simulink model "Generic_sedan"  (R2023b)
settings: Solver=VariableStepAuto  StartTime=0.0  StopTime=26  FixedStep=0.001  MaxStep=0.01  RelTol=1e-4
InitFcn:
  | A = readmatrix(['data' filesep 'A.dat']);
  | B = readmatrix(['data' filesep 'B.dat']);
  | C = readmatrix(['data' filesep 'C.dat']);
  | D = readmatrix(['data' filesep 'D.dat']);
  | 
  | Z0 = readmatrix(['data' filesep 'Z0.dat']);
  | m = readmatrix(['data' filesep 'mass.dat']);
  | IG = readmatrix(['data' filesep 'IG.dat']);
  | 
  | z = readmatrix(['data' filesep 'z.dat']);
  | l = readmatrix(['data' filesep 'l.dat']);
  | fbf = readmatrix(['data' filesep 'brake.dat']);
libraries: simulink x10, matrix_library x2, slpidlib x1
(part 1 of 2)
settings Model: Creator=minaker  LastModifiedBy=minaker
settings SimscapeCC: EditingMode=Restricted

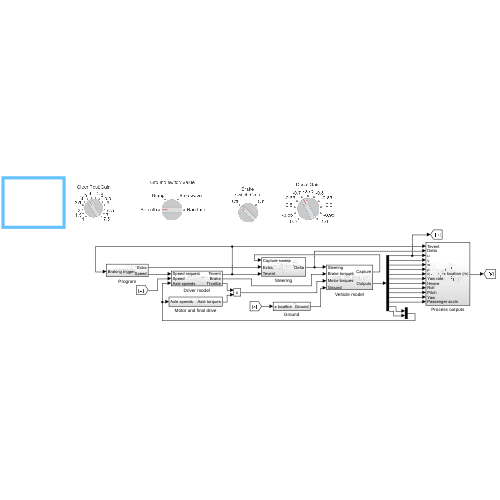
[thumbnail: Simulink's stored preview of the top-level diagram]
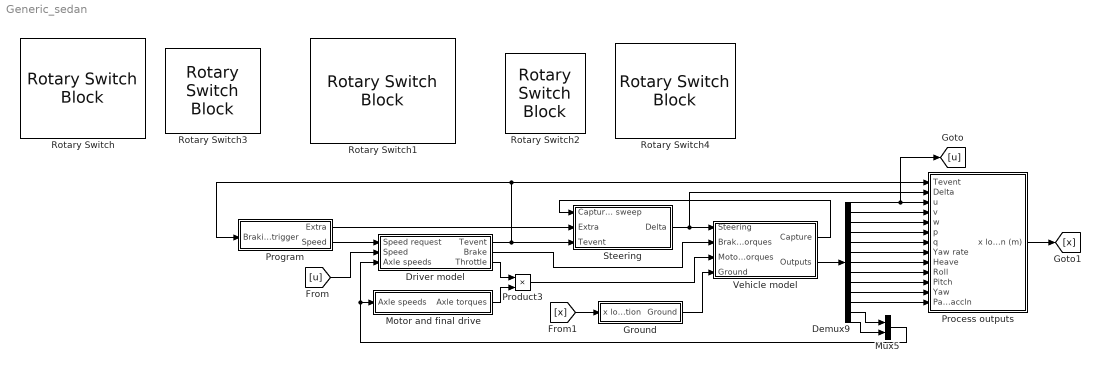
== system Generic_sedan ==
  Demux9 : Demux  Outputs=13
  Driver model : Subsystem
  Ground : Subsystem
  Motor and final drive : Subsystem
  Mux5 : Mux  Inputs=2
  Process outputs : Subsystem
  Product3 : Product
  Program : Subsystem
  Rotary Switch{,1..4} (5 alike) : RotarySwitchBlock
  Steering : Subsystem
  Vehicle model : Subsystem
  wires:
  Product3/1 -> Vehicle model/3(Motor torques)
  Vehicle model/2(Outputs) -> Demux9/1
  Demux9/12 -> Mux5/1
  Demux9/13 -> Mux5/2
  Motor and final drive/1(Axle torques) -> Product3/2
  Demux9/2 -> Process outputs/4(v)
  Demux9/1 -> [u], Process outputs/3(u)
  Demux9/10 -> Process outputs/12(Yaw)
  Driver model/2(Brake) -> Vehicle model/2(Brake torques)
  Driver model/3(Throttle) -> Product3/1
  Demux9/6 -> Process outputs/8(Yaw rate)
  Demux9/8 -> Process outputs/10(Roll)
  Demux9/9 -> Process outputs/11(Pitch)
  Demux9/7 -> Process outputs/9(Heave)
  Demux9/11 -> Process outputs/13(Passenger accln)
  Steering/1(Delta) -> Process outputs/2(Delta), Vehicle model/1(Steering)
  Vehicle model/1(Capture) -> Steering/1(Capture sweep)
  Demux9/3 -> Process outputs/5(w)
  Demux9/4 -> Process outputs/6(p)
  Demux9/5 -> Process outputs/7(q)
  [u] -> Driver model/2(Speed)
  Process outputs/1(x location (m)) -> [x]
  Driver model/1(Tevent) -> Program/1(Braking trigger), Process outputs/1(Tevent), Steering/3(Tevent)
  Mux5/1 -> Driver model/3(Axle speeds), Motor and final drive/1(Axle speeds)
  Program/1(Extra) -> Steering/2(Extra)
  Program/2(Speed) -> Driver model/1(Speed request)
  [x] -> Ground/1(x location)
  Ground/1(Ground) -> Vehicle model/4(Ground)

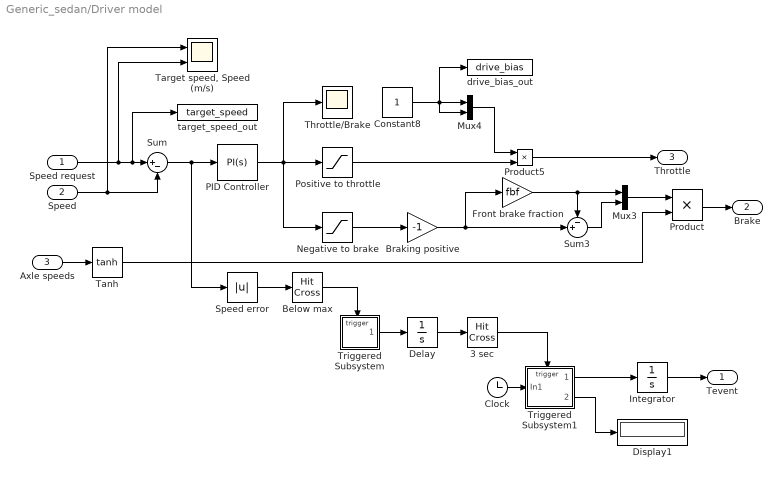
== system Generic_sedan/Driver model ==
  Speed request : Inport
  Speed : Inport  Port=2
  Axle speeds : Inport  Port=3
  3 sec : HitCross  HitCrossingOffset=3  HitCrossingDirection=rising
  Below max : HitCross  HitCrossingOffset=0.1  HitCrossingDirection=falling
  Braking positive : Gain  Gain=-1
  Clock : Clock
  Constant8 : Constant
  Delay : Integrator
  Display1 : Display
  Front brake fraction : Gain  Gain=fbf
  Integrator : Integrator
  Mux3 : Mux  Inputs=2
  Mux4 : Mux  Inputs=2
  Negative to brake : Saturate  UpperLimit=0  LowerLimit=-Inf
  PID Controller : slpidlib/PID Controller  Controller=PI  Form=Parallel  TimeDomain=Continuous-time  UseExternalTs=off  SampleTime=-1  IntegratorMethod=Forward Euler  FilterMethod=Forward Euler  ControllerParametersSource=internal  P=0.75  I=0.0075  UseKiTs=off  D=0.2  N=100  UseFilter=on  TunerSelectOption=Transfer Function Based (PID Tuner App)  InitialConditionSource=internal  InitialConditionForIntegrator=0  InitialConditionForFilter=0  DifferentiatorICPrevScaledInput=0  ExternalReset=none  TrackingMode=off  Kt=1  LimitOutput=on  SatLimitsSource=internal  UpperSaturationLimit=1  LowerSaturationLimit=-1  LinearizeAsGain=on  AntiWindupMode=clamping  Kb=1  LimitIntegrator=off  UpperIntegratorSaturationLimit=inf  LowerIntegratorSaturationLimit=-inf  POutMin=[]  POutMax=[]  IOutMin=[]  IOutMax=[]  DOutMin=[]  DOutMax=[]  NOutMin=[]  NOutMax=[]  SumOutMin=[]  SumOutMax=[]  SaturationOutMin=[]  SaturationOutMax=[]  PParamMin=[]  PParamMax=[]  IParamMin=[]  IParamMax=[]  DParamMin=[]  DParamMax=[]  NParamMin=[]  NParamMax=[]  KbParamMin=[]  KbParamMax=[]  KtParamMin=[]  KtParamMax=[]  KbOutMin=[]  KbOutMax=[]  KtOutMin=[]  KtOutMax=[]  IntegratorOutMin=[]  IntegratorOutMax=[]  FilterOutMin=[]  FilterOutMax=[]  SumI1OutMin=[]  SumI1OutMax=[]  SumI2OutMin=[]  SumI2OutMax=[]  SumI3OutMin=[]  SumI3OutMax=[]  SumI4OutMin=[]  SumI4OutMax=[]  SumDOutMin=[]  SumDOutMax=[]  DifferentiatorOutMin=[]  DifferentiatorOutMax=[]  FilterDiffOutCoefMin=[]  FilterDiffOutCoefMax=[]  ReciprocalOutMin=[]  ReciprocalOutMax=[]  SumDenOutMin=[]  SumDenOutMax=[]  SumNumOutMin=[]  SumNumOutMax=[]  DivideOutMin=[]  DivideOutMax=[]  UdiffTsProdOutMin=[]  UdiffTsProdOutMax=[]  NTsProdOutMin=[]  NTsProdOutMax=[]  UintegralTsProdOutMin=[]  UintegralTsProdOutMax=[]  UngainTsProdOutMin=[]  UngainTsProdOutMax=[]  ClampingZeroOutDataTypeStr=Inherit: Inherit via back propagation  ClampingZeroOutMin=[]  ClampingZeroOutMax=[]  FilterDenConstantOutDataTypeStr=Inherit: Inherit via back propagation  FilterDenConstantOutMin=[]  FilterDenConstantOutMax=[]  PCopyOutDataTypeStr=Inherit: Inherit via back propagation  PCopyOutMin=[]  PCopyOutMax=[]  NCopyOutDataTypeStr=Inherit: Inherit via back propagation  NCopyOutMin=[]  NCopyOutMax=[]  IntegratorContinuousStateAttributes=''  IntegratorStateMustResolveToSignalObject=off  IntegratorRTWStateStorageClass=Auto  FilterContinuousStateAttributes=''  FilterStateMustResolveToSignalObject=off  FilterRTWStateStorageClass=Auto  ParallelPVariant=InternalParameters  IdealPVariant=Disabled  IVariant=InternalParameters  DVariant=Disabled  IntegratorVariant=Continuous  SatVariant=Enabled  AWVariant=ContClampingParallel  PCopyVariant=Disabled  TRVariant=Disabled  FdbkBlocksVariant=Forward  IdealPFdbkVariant=Disabled  SatFdbkVariant=Disabled  DerivativeFilterVariant=Disabled  NVariant=Disabled  NCopyVariant=Disabled_SignalSpec  FilterICVariant=Disabled  IntegratorICVariant=InternalICs  ExternalResetVariant=Disabled  TRSumVariant=Passthrough  SumFdbkVariant=Disabled  SumVariant=Sum_PI  TsampFilterVariant=InternalTs  TsampNgainVariant=Passthrough  TsampIntegralVariant=Disabled_SignalSpec  ExternalSaturationOutDataTypeStr=Inherit: Same as second input
  Positive to throttle : Saturate  UpperLimit=Inf  LowerLimit=0
  Product : Product
  Product5 : Product
  Speed error : Abs  SaturateOnIntegerOverflow=off
  Sum : Sum  Inputs=|+-
  Sum3 : Sum  Inputs=-+|
  Tanh : Trigonometry  Operator=tanh
  "Target speed, Speed (m/s)" : Scope  NumInputPorts=2
  Throttle/Brake : Scope
  Triggered Subsystem : Subsystem  TreatAsAtomicUnit=on
  Triggered Subsystem1 : Subsystem  TreatAsAtomicUnit=on
  drive_bias_out : ToWorkspace  VariableName=drive_bias  SaveFormat=Timeseries  SampleTime=-1
      settings: Decimation=3
  target_speed_out : ToWorkspace  VariableName=target_speed  SaveFormat=Timeseries  SampleTime=-1
      settings: Decimation=3
  Tevent : Outport
  Brake : Outport  Port=2
  Throttle : Outport  Port=3
  wires:
  Product5/1 -> Throttle/1
  Speed/1 -> "Target speed, Speed (m/s)"/1, Sum/2
  Mux4/1 -> Product5/1
  Positive to throttle/1 -> Product5/2
  Constant8/1 -> drive_bias_out/1, Mux4/1, Mux4/2
  PID Controller/1 -> Throttle/Brake/1, Negative to brake/1, Positive to throttle/1
  Braking positive/1 -> Front brake fraction/1, Sum3/2
  Speed request/1 -> target_speed_out/1, Sum/1, "Target speed, Speed (m/s)"/2
  Sum3/1 -> Mux3/2
  Front brake fraction/1 -> Mux3/1, Sum3/1
  Negative to brake/1 -> Braking positive/1
  Mux3/1 -> Product/1
  Sum/1 -> Speed error/1, PID Controller/1
  Speed error/1 -> Below max/1
  Triggered Subsystem/1(Out1) -> Delay/1
  Below max/1 -> Triggered Subsystem/Trigger
  3 sec/1 -> Triggered Subsystem1/Trigger
  Delay/1 -> 3 sec/1
  Triggered Subsystem1/1(Out1) -> Integrator/1
  Triggered Subsystem1/2(Start time) -> Display1/1
  Clock/1 -> Triggered Subsystem1/1(In1)
  Integrator/1 -> Tevent/1
  Tanh/1 -> Product/2
  Axle speeds/1 -> Tanh/1
  Product/1 -> Brake/1

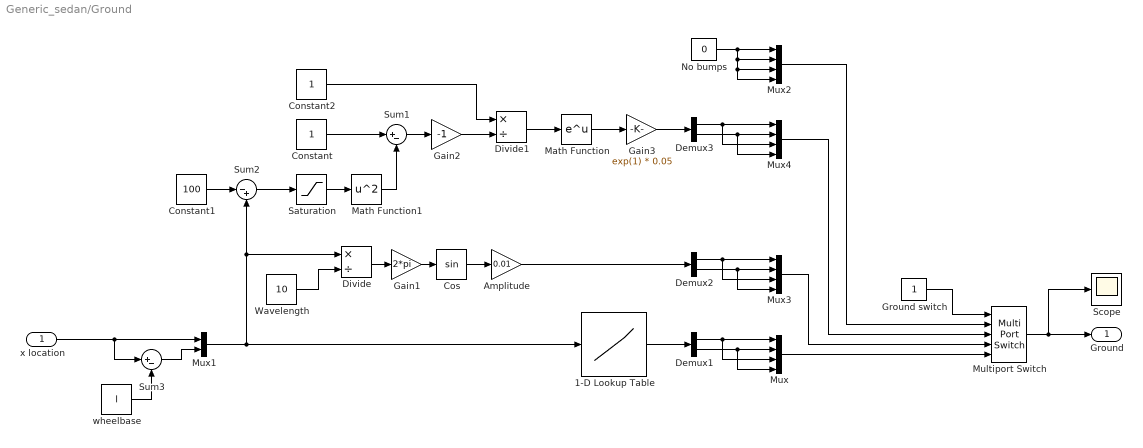
== system Generic_sedan/Ground ==
  x location : Inport
  1-D Lookup Table : Lookup_n-D  NumberOfTableDimensions=1  BreakpointsForDimension1=z(:,1)  Table=z(:,2)  ExtrapMethod=Clip  InternalRulePriority=Speed  RndMeth=Simplest
  Amplitude : Gain  Gain=0.01
  Constant : Constant
  Constant1 : Constant  Value=100
  Constant2 : Constant
  Cos : Trigonometry
  Demux1 : Demux  Outputs=2
  Demux2 : Demux  Outputs=2
  Demux3 : Demux  Outputs=2
  Divide : Product  Inputs=*/
  Divide1 : Product  Inputs=*/
  Gain1 : Gain  Gain=2*pi
  Gain2 : Gain  Gain=-1
  Gain3 : Gain  Gain=exp(1) * 0.05
  Ground switch : Constant
  Math Function : Math
  Math Function1 : Math  Operator=square
  Multiport Switch : MultiPortSwitch  Inputs=4  SaturateOnIntegerOverflow=off  InputSameDT=off
  Mux{,2..4} (4 alike) : Mux
  Mux1 : Mux  Inputs=2
  No bumps : Constant  Value=0
  Saturation : Saturate  UpperLimit=1  LowerLimit=-1
  Scope : Scope
  Sum1 : Sum  Inputs=|+-
  Sum2 : Sum  Inputs=|-+
  Sum3 : Sum  Inputs=|+-
  Wavelength : Constant  Value=10
  wheelbase : Constant  Value=l
  Ground : Outport
  wires:
  Mux2/1 -> Multiport Switch/2
  Multiport Switch/1 -> Scope/1, Ground/1
  Demux1/2 -> Mux/4, Mux/2
  Demux1/1 -> Mux/3, Mux/1
  wheelbase/1 -> Sum3/2
  Sum3/1 -> Mux1/2
  1-D Lookup Table/1 -> Demux1/1
  Ground switch/1 -> Multiport Switch/1
  Mux/1 -> Multiport Switch/5
  x location/1 -> Sum3/1, Mux1/1
  No bumps/1 -> Mux2/3, Mux2/4, Mux2/2, Mux2/1
  Amplitude/1 -> Demux2/1
  Mux1/1 -> Divide/1, Sum2/2, 1-D Lookup Table/1
  Demux2/2 -> Mux3/4, Mux3/2
  Demux2/1 -> Mux3/3, Mux3/1
  Mux3/1 -> Multiport Switch/4
  Divide/1 -> Gain1/1
  Gain1/1 -> Cos/1
  Wavelength/1 -> Divide/2
  Cos/1 -> Amplitude/1
  Gain2/1 -> Divide1/2
  Divide1/1 -> Math Function/1
  Constant/1 -> Sum1/1
  Math Function1/1 -> Sum1/2
  Sum1/1 -> Gain2/1
  Saturation/1 -> Math Function1/1
  Constant1/1 -> Sum2/1
  Sum2/1 -> Saturation/1
  Math Function/1 -> Gain3/1
  Constant2/1 -> Divide1/1
  Gain3/1 -> Demux3/1
  Demux3/1 -> Mux4/3, Mux4/1
  Demux3/2 -> Mux4/4, Mux4/2
  Mux4/1 -> Multiport Switch/3

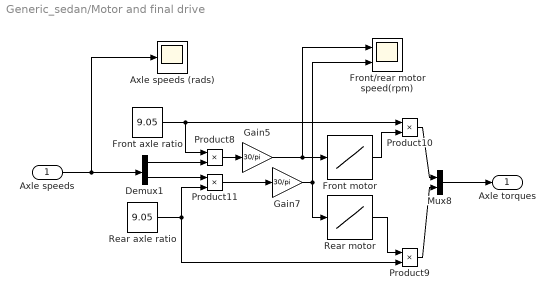
== system Generic_sedan/Motor and final drive ==
  Axle speeds : Inport
  Axle speeds (rads) : Scope
  Demux1 : Demux  Outputs=2
  Front axle ratio : Constant  Value=9.05
  Front motor : Lookup_n-D  NumberOfTableDimensions=1  BreakpointsForDimension1=[0;50;100;150;200;250;300;350;400;450;500;550;600;650;700;750;800;850;900;950;1000;1050;1100;1150;1200;1250;1300;1350;1400;1450;1500;1550;1600;1650;1700;1750;1800;1850;1900;1950;2000;2050;2100;2150;2200;2250;2300;2350;2400;2450;2500;2550;2600;2650;2700;2750;2800;2850;2900;2950;3000;3050;3100;3150;3200;3250;3300;3350;3400;3450;3500;3550;3600;3650;3700;3750;3800;3850;3900;3950;4000;4050;4100;4150;4200;4250;4300;4350;4400;4450;4500;4550;4600;4650;4700;4750;4800;4850;4900;4950;5000;5050;5100;5150;5200;5250;5300;5350;5400;5450;5500;5550;5600;5650;5700;5750;5800;5850;5900;5950;6000;6050;6100;6150;6200;6250;6300;6350;6400;6450;6500;6550;6600;6650;6700;6750;6800;6850;6900;6950;7000;7050;7100;7150;7200;7250;7300;7350;7400;7450;7500;7550;7600;7650;7700;7750;7800;7850;7900;7950;8000;8050;8100;8150;8200;8250;8300;8350;8400;8450;8500;8550;8600;8650;8700;8750;8800;8850;8900;8950;9000;9050;9100;9150;9200;9250;9300;9350;9400;9450;9500;9550;9600;9650;9700;9750;9800;9850;9900;9950;10000;10050;10100;10150;10200;10250;10300;10350;10400;10450;10500;10550;10600;10650;10700;10750;10800;10850;10900;10950;11000;11050;11100;11150;11200;11250;11300;11350;11400;11450;11500;11550;11600;11650;11700;11750;11800;11850;11900;11950;12000;12050;12100;12150;12200;12250;12300;12350;12400;12450;12500;12550;12600;12650;12700;12750;12800;12850;12900;12950;13000;13050;13100;13150;13200;13250;13300;13350;13400;13450;13500;13550;13600;13650;13700;13750;13800]  Table=[151.278471649211;150.863507782483;150.857645204683;150.851798439641;150.845961214183;150.840130739586;150.834305445898;150.828484331262;150.822666703624;150.816852057881;150.811040010119;150.805230259282;150.799422563368;150.793616723888;150.787812575288;150.782009977530;150.776208810713;150.770408971108;150.764610368151;150.758812922132;150.753016562399;150.747221225919;150.741426856141;150.735633402060;150.729840817460;150.724049060281;150.718258092094;150.712467877664;150.706678384571;150.700889582896;150.695101444949;150.689313945031;150.683527059236;150.677740765271;150.671955042299;150.666169870810;150.660385232498;150.654601110154;150.648817487573;150.643034349475;150.637251681422;150.631469469760;150.625687701550;150.619906364522;150.614125447022;150.608344937967;150.602564826808;150.596785103490;150.591005758422;150.585226782442;150.579448166795;150.573669903103;150.567891983343;150.562114399825;150.556337145175;150.550560212312;150.544783594433;150.539007284998;150.533231277717;150.527455566531;150.521680145605;150.515905009314;150.510130152233;150.504355569124;150.498581254931;148.374181079972;146.125974258770;143.945037424496;141.828191440898;139.772684341068;137.775894243506;135.835157562690;133.948829662349;132.113904887137;130.328575497099;128.590978243296;126.898873510717;125.250831781071;123.645086677358;122.079845291043;120.553855681789;119.065531893495;117.613516943143;116.196631674882;114.813197353996;113.462607953756;112.143116898742;110.854289029982;109.594402325692;108.362997543078;107.158884499023;105.981325021586;104.829358289475;103.702163956374;102.598944505611;101.518963997732;100.461458577429;99.4257696628103;98.4112032057036;97.4169803632393;96.4428468494649;95.4879934255911;94.5519655023934;93.6336039738249;92.7339362228427;91.8503667621564;90.9842571556953;90.1335231457530;89.2993699380107;88.4796659256438;87.6757465870287;86.8854186202727;86.1095497053428;85.3480053387293;84.5988715272067;83.8638251758735;83.1403184969489;82.4296640384837;81.7310399176694;81.0447873302831;80.3688805105759;79.7051959749083;79.0517449603443;78.4086231766840;77.7762824954103;77.1545523243600;76.5415929088006;75.9390023745799;75.3457153739749;74.7616213898289;74.1870080607537;73.6201508895266;73.0629516796206;72.5131001669698;71.9719338669643;71.4393535756975;70.9134865309499;70.3963184515362;69.8864581840491;69.3829019088306;68.8873785972233;68.3994010157060;67.9178864974784;67.4421538676144;66.9737815819947;66.5124360742594;66.0562807895463;65.6074841358173;65.1635947359257;64.7268069675545;64.2947231500399;63.8694815701027;63.4487227952091;63.0345689138391;62.6255122413869;62.2206415044942;61.8223298316254;61.4279939494809;61.0397435640339;60.6561280103982;60.2761819776827;59.9023223995399;59.5328468246745;59.1667632052020;58.8065098220250;58.4504077906492;58.0974490866022;57.7500709024121;57.4066274669585;57.0660939915105;56.7309147606174;56.3994683410035;56.0707202646022;55.7471069493456;55.4262052260204;55.1099727704398;54.7971666570846;54.4867411788298;54.1811164617496;53.8787500903933;53.5795924172299;53.2825709746378;52.9902784666275;52.7010368836716;52.4137990680552;52.1309413888743;51.8509908230479;51.5739038180854;51.2985649381260;51.0275936092540;50.7593508293397;50.4927991289585;50.2302556320192;49.9703169896832;49.7119478679885;49.4574468745715;49.2054333900219;48.9558725933389;48.7076241958030;48.4632837399324;48.2212850899552;47.9815973534268;47.7430784882541;47.5082121649214;47.2756519874389;47.0442958892288;46.8163352461487;46.5904893858102;46.3667271851825;46.1439110744480;45.9245721439951;45.7072299260645;45.4918575830820;45.2773233799879;45.0661281374574;44.8568211134734;44.6493778189262;44.4437738063396;44.2387987606263;44.0371626899314;43.8372897474568;43.6391585877190;43.4416546749887;43.2472080094171;43.0544327298518;42.8633080852959;42.6738128625357;42.4847391415345;42.2987511504260;42.1143278668312;41.9314509531562;41.7501004959835;41.5690724994407;41.3910035521333;41.2144025457871 ...(+714 chars)]  InternalRulePriority=Speed  RndMeth=Simplest
  Front/rear motor speed(rpm) : Scope  NumInputPorts=2
  Gain5 : Gain  Gain=30/pi
  Gain7 : Gain  Gain=30/pi
  Mux8 : Mux  Inputs=2
  Product{8..11} (4 alike) : Product
  Rear axle ratio : Constant  Value=9.05
  Rear motor : Lookup_n-D  NumberOfTableDimensions=1  BreakpointsForDimension1=[0;50;100;150;200;250;300;350;400;450;500;550;600;650;700;750;800;850;900;950;1000;1050;1100;1150;1200;1250;1300;1350;1400;1450;1500;1550;1600;1650;1700;1750;1800;1850;1900;1950;2000;2050;2100;2150;2200;2250;2300;2350;2400;2450;2500;2550;2600;2650;2700;2750;2800;2850;2900;2950;3000;3050;3100;3150;3200;3250;3300;3350;3400;3450;3500;3550;3600;3650;3700;3750;3800;3850;3900;3950;4000;4050;4100;4150;4200;4250;4300;4350;4400;4450;4500;4550;4600;4650;4700;4750;4800;4850;4900;4950;5000;5050;5100;5150;5200;5250;5300;5350;5400;5450;5500;5550;5600;5650;5700;5750;5800;5850;5900;5950;6000;6050;6100;6150;6200;6250;6300;6350;6400;6450;6500;6550;6600;6650;6700;6750;6800;6850;6900;6950;7000;7050;7100;7150;7200;7250;7300;7350;7400;7450;7500;7550;7600;7650;7700;7750;7800;7850;7900;7950;8000;8050;8100;8150;8200;8250;8300;8350;8400;8450;8500;8550;8600;8650;8700;8750;8800;8850;8900;8950;9000;9050;9100;9150;9200;9250;9300;9350;9400;9450;9500;9550;9600;9650;9700;9750;9800;9850;9900;9950;10000;10050;10100;10150;10200;10250;10300;10350;10400;10450;10500;10550;10600;10650;10700;10750;10800;10850;10900;10950;11000;11050;11100;11150;11200;11250;11300;11350;11400;11450;11500;11550;11600;11650;11700;11750;11800;11850;11900;11950;12000;12050;12100;12150;12200;12250;12300;12350;12400;12450;12500;12550;12600;12650;12700;12750;12800;12850;12900;12950;13000;13050;13100;13150;13200;13250;13300;13350;13400;13450;13500;13550;13600;13650;13700;13750;13800]  Table=[432.243928408188;430.974439582432;430.956179022406;430.937971427874;430.919796209269;430.901644104877;430.883509858563;430.865390095315;430.847282471915;430.829185270798;430.811097181604;430.793017173390;430.774944414988;430.756878222831;430.738818025389;430.720763338111;430.702713745266;430.684668886477;430.666628446533;430.648592147528;430.630559742721;430.612531011656;430.594505756247;430.576483797589;430.558464973357;430.540449135636;430.522436149121;430.504425889595;430.486418242650;430.468413102584;430.450410371463;430.432409958315;430.414411778418;430.396415752698;430.378421807187;430.360429872554;430.342439883693;430.324451779352;430.306465501809;430.288480996581;430.270498212163;430.252517099794;430.234537613252;430.216559708658;430.198583344313;430.180608480534;430.162635079523;430.144663105232;430.126692523248;430.108723300689;430.090755406101;430.072788809376;430.054823481660;430.036859395286;430.018896523699;430.000934841393;429.982974323852;429.965014947491;429.947056689611;429.929099528346;429.911143442620;429.893188412107;429.875234417191;429.857281438932;429.839329459032;429.821378459799;427.981721433497;421.593724980700;415.393957153120;409.373720022615;403.525491314955;397.842014747280;392.316393278445;386.942169399268;381.713191334335;376.622937315821;371.667497699383;366.841160078948;362.137730929994;357.553828148806;353.084910683754;348.725261434143;344.472711529334;340.322323403211;336.270778863834;332.314595712636;328.450457205214;324.675146866800;320.985637221670;317.379016616004;313.852538681236;310.403848313197;307.030644702009;303.729239788566;300.498074173125;297.334940004498;294.237701043453;291.204256508991;288.232850000853;285.321365981808;282.468192927640;279.671478179448;276.929600964921;274.240964075862;271.604031735127;269.017326671512;266.479427359743;263.988965414691;261.544623132608;259.145131165270;256.789266322546;254.475849492834;252.203743675887;249.971852119045;247.779116552168;245.624515514459;243.507062767986;241.425805792333;239.379824355837;237.368229158974;235.390160545651;233.444787397876;231.531305336144;229.648936957453;227.796929383204;225.974553870265;224.181104888187;222.415899192137;220.678274919441;218.967590603395;217.283224394710;215.624573747959;213.991054310818;212.382098840968;210.797157691598;209.235697164105;207.697199156691;206.181161134820;204.687094611862;203.214525470400;201.762992987159;200.332049501511;198.921260102066;197.530202106113;196.158464161338;194.805646820932;193.471361175082;192.155229003378;190.856882259308;189.575962937981;188.312122535456;187.065021661250;185.834329552786;184.619725127149;183.420894478029;182.237532335583;181.069341668332;179.916031372645;178.777319974436;177.652931593355;176.542597603395;175.446056040499;174.363051394840;173.293334410585;172.236661892536;171.192796519340;170.161506663305;169.142566215623;168.135754417792;167.140855698028;166.157659512809;165.186077775014;164.225693601322;163.276412134865;162.338041949438;161.410395996382;160.493291527820;159.586549792313;158.689996323496;157.803460118424;156.926773874417;156.059775120300;155.202303824061;154.354203797618;153.515322248111;152.685509686281;151.864619837427;151.052509555544;150.249038739976;149.454070254761;148.667469850468;147.889106088577;147.118850267707;146.356576352747;145.602160905490;144.855483017336;144.116424244760;143.384868544377;142.660702212323;141.943813822632;141.234094168514;140.531436203406;139.835734983580;139.146887610424;138.464793172002;137.789352685506;137.120469035850;136.458046910424;135.801992734899;135.152214593453;134.508622146712;133.871126584102;133.239713675600;132.614175112303;131.994482703112;131.380554873391;130.772311558861;130.169674170608;129.572565560543;128.980909988777;128.394633087277;127.813661829509;127.237924489186;126.667350600028;126.101870893083;125.541417204238;124.985922291029;124.435319446649;123.889541580428;123.348555891353;122.812257815484;122.280602993833;121.753531285584;121.230982638504;120.712902960770 ...(+714 chars)]  InternalRulePriority=Speed  RndMeth=Simplest
  Axle torques : Outport
  wires:
  Front axle ratio/1 -> Product10/1, Product8/1
  Mux8/1 -> Axle torques/1
  Axle speeds/1 -> Demux1/1, Axle speeds (rads)/1
  Product8/1 -> Gain5/1
  Product10/1 -> Mux8/1
  Demux1/2 -> Product11/1
  Gain7/1 -> Rear motor/1, Front/rear motor speed(rpm)/2
  Rear axle ratio/1 -> Product9/2, Product11/2
  Demux1/1 -> Product8/2
  Rear motor/1 -> Product9/1
  Product11/1 -> Gain7/1
  Product9/1 -> Mux8/2
  Gain5/1 -> Front/rear motor speed(rpm)/1, Front motor/1
  Front motor/1 -> Product10/2

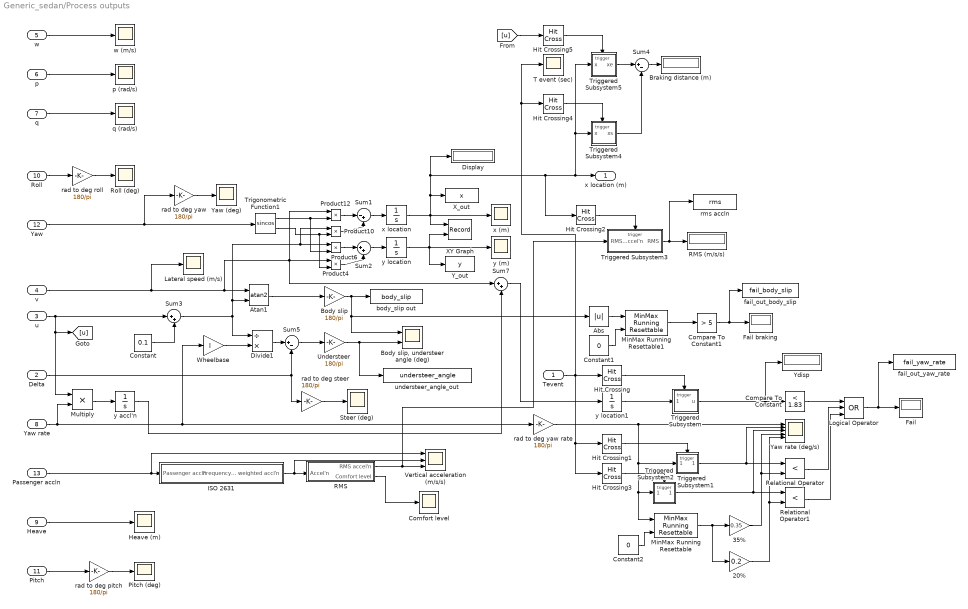
== system Generic_sedan/Process outputs ==
  Tevent : Inport
  Delta : Inport  Port=2
  u : Inport  Port=3
  v : Inport  Port=4
  w : Inport  Port=5
  p : Inport  Port=6
  q : Inport  Port=7
  Yaw rate : Inport  Port=8
  Heave : Inport  Port=9
  Roll : Inport  Port=10
  Pitch : Inport  Port=11
  Yaw : Inport  Port=12
  Passenger accln : Inport  Port=13
  20% : Gain  Gain=0.2
  35% : Gain  Gain=0.35
  Abs : Abs  SaturateOnIntegerOverflow=off
  Atan1 : Trigonometry  Operator=atan2
  Body slip : Gain  Gain=180/pi
  "Body slip, understeer angle (deg)" : Scope  NumInputPorts=2
  Braking distance (m) : Display
  Comfort level : Scope
  Compare To Constant : simulink/Logic and Bit Operations/Compare To Constant  relop=<  const=1.83  OutDataTypeStr=boolean
  Compare To Constant1 : simulink/Logic and Bit Operations/Compare To Constant  relop=>  const=5  OutDataTypeStr=boolean
  Constant : Constant  Value=0.1
  Constant1 : Constant  Value=0  OutDataTypeStr=boolean
  Constant2 : Constant  Value=0  OutDataTypeStr=boolean
  Display : Display
  Divide1 : Product  Inputs=/*
  Fail : Display
  Fail braking : Display
  Heave (m) : Scope
  Hit Crossing : HitCross  HitCrossingOffset=0.75/0.7  HitCrossingDirection=rising
  Hit Crossing1 : HitCross  HitCrossingOffset=1/0.7+0.5+1  HitCrossingDirection=rising
  Hit Crossing2 : HitCross  HitCrossingOffset=500  HitCrossingDirection=rising
  Hit Crossing3 : HitCross  HitCrossingOffset=1/0.7+0.5+1.75  HitCrossingDirection=rising
  Hit Crossing4 : HitCross  HitCrossingOffset=1e-6  HitCrossingDirection=rising
  Hit Crossing5 : HitCross  HitCrossingOffset=8/3.6  HitCrossingDirection=falling
  ISO 2631 : Subsystem
  Lateral speed (m/s) : Scope
  Logical Operator : Logic  Operator=OR  Inputs=3  AllPortsSameDT=off  OutDataTypeStr=boolean
  MinMax Running Resettable : simulink/Math Operations/MinMax Running Resettable  Function=min  vinit=0.0
  MinMax Running Resettable1 : simulink/Math Operations/MinMax Running Resettable  Function=max  vinit=0.0
  Multiply : Product  Inputs=**
  Pitch (deg) : Scope
  Product{4,6,10,12} (4 alike) : Product
  RMS : Subsystem
  RMS (m/s/s) : Display
  Relational Operator : RelationalOperator  Operator=<  OutDataTypeStr=boolean  RndMeth=Simplest  InputSameDT=off
  Relational Operator1 : RelationalOperator  Operator=<  OutDataTypeStr=boolean  RndMeth=Simplest  InputSameDT=off
  Roll (deg) : Scope
  Steer (deg) : Scope
  Sum1 : Sum  Inputs=|-+
  Sum2 : Sum  Inputs=|++
  Sum3 : Sum  Inputs=|++
  Sum4 : Sum  Inputs=|+-
  Sum5 : Sum  Inputs=|+-
  Sum7 : Sum  Inputs=|++
  T event (sec) : Scope
  Triggered Subsystem : Subsystem  TreatAsAtomicUnit=on
  Triggered Subsystem1 : Subsystem  TreatAsAtomicUnit=on
  Triggered Subsystem2 : Subsystem  TreatAsAtomicUnit=on
  Triggered Subsystem3 : Subsystem  TreatAsAtomicUnit=on
  Triggered Subsystem4 : Subsystem  TreatAsAtomicUnit=on
  Triggered Subsystem5 : Subsystem  TreatAsAtomicUnit=on
  Trigonometric Function1 : Trigonometry  Operator=sincos
  Understeer : Gain  Gain=180/pi
  Vertical acceleration (m/s/s) : Scope  NumInputPorts=3
  Wheelbase : Gain  Gain=l
  XY Graph : Record  FileSettingsInternal="{\"entries\":[{\"content\":{\"excelSettings\":{\"content\":{},\"type\":\"Streamout.ExcelSettings\"}},\"type\":\"Streamout.FileSettingStorage\",\"uuid\":\"\"}],\"packageUris\":[\"http:\\/\\/schema.mathworks.com\\/mf0\\/streamout_blocks\\/R2020a\"],\"version\":\"1.0\"}"  Layout=[1 1]  SignalsInternal="{\"entries\":[{\"content\":{\"signals\":[{\"content\":{\"blockPath\":[],\"dimensions\":[1],\"domain\":\"\",\"lineColor\":\"#7e2f8e\",\"plots\":[1],\"port\":1,\"sid\":[\"\"],\"signalID\":3805,\"signalName\":\"x location\"},\"type\":\"RecordBlkView.Signal\",\"uuid\":\"\"},{\"content\":{\"blockPath\":[],\"dimensions\":[1],\"domain\":\"\",\"lineColor\":\"#77ac30\",\"plots\":[1],\"port\":2,\"sid\":[\"\"],\"signalID\":3809,\"signalName\":\"y location\"},\"type\":\"RecordBlkView.Signal\",\"uuid\":\"\"}]},\"type\":\"RecordBlkView.InputSignals\",\"uuid\":\"\"}],\"packageUris\":[\"http:\\/\\/schema.mathworks.com\\/mf0\\/streamout_blocks\\/R2020a\"],\"version\":\"1.0\"}"  VisualizationBindings="{\"xyplotplugin\":{\"info\":[{\"series\":[{\"bindingParametersList\":[{\"parameter\":\"X-Axis\",\"signalID\":3805,\"signalName\":\"x location\"},{\"parameter\":\"Y-Axis\",\"signalID\":3809,\"signalName\":\"y location\"}],\"seriesID\":11048}],\"subplotID\":1}]}}"  CompatibilityTag=XY
  X_out : ToWorkspace  VariableName=x  SaveFormat=Timeseries  SampleTime=-1
      settings: Decimation=3
  Y_out : ToWorkspace  VariableName=y  SaveFormat=Timeseries  SampleTime=-1
      settings: Decimation=3
  Yaw (deg) : Scope
  Yaw rate (deg/s) : Scope  NumInputPorts=5
  Ydisp : Display
  body_slip out : ToWorkspace  VariableName=body_slip  SaveFormat=Timeseries  SampleTime=-1
      settings: Decimation=3
  fail_out_body_slip : ToWorkspace  VariableName=fail_body_slip  SaveFormat=Timeseries  SampleTime=-1
      settings: Decimation=3
  fail_out_yaw_rate : ToWorkspace  VariableName=fail_yaw_rate  SaveFormat=Timeseries  SampleTime=-1
      settings: Decimation=3
  p (rad/s) : Scope
  q (rad/s) : Scope
  rad to deg pitch : Gain  Gain=180/pi
  rad to deg roll : Gain  Gain=180/pi
  rad to deg steer : Gain  Gain=180/pi
  rad to deg yaw : Gain  Gain=180/pi
  rad to deg yaw rate : Gain  Gain=180/pi
  rms accln : ToWorkspace  VariableName=rms  SaveFormat=Timeseries  SampleTime=-1
      settings: Decimation=3
  understeer_angle_out : ToWorkspace  VariableName=understeer_angle  SaveFormat=Timeseries  SampleTime=-1
      settings: Decimation=3
  w (m/s) : Scope
  x (m) : Scope
  x location : Integrator
  y (m) : Scope
  y accl'n : Integrator
  y location : Integrator
  y location1 : Integrator
  x location (m) : Outport
  wires:
  Sum2/1 -> y location/1
  Product10/1 -> Sum1/2
  Divide1/1 -> Sum5/1
  Wheelbase/1 -> Divide1/2
  Delta/1 -> rad to deg steer/1, Sum5/2
  Body slip/1 -> "Body slip, understeer angle (deg)"/1, Abs/1, body_slip out/1
  Trigonometric Function1/2 -> Product10/2, Product4/2
  Trigonometric Function1/1 -> Product12/2, Product6/2
  Sum1/1 -> x location/1
  Sum3/1 -> Divide1/1, Product10/1, Product6/1, Atan1/2
  Yaw/1 -> rad to deg yaw/1, Trigonometric Function1/1
  Product4/1 -> Sum2/2
  Product6/1 -> Sum2/1
  Sum5/1 -> Understeer/1
  Product12/1 -> Sum1/1
  Understeer/1 -> "Body slip, understeer angle (deg)"/2, understeer_angle_out/1
  Atan1/1 -> Body slip/1
  y location/1 -> Y_out/1, y (m)/1, XY Graph/2
  rad to deg pitch/1 -> Pitch (deg)/1
  Heave/1 -> Heave (m)/1
  rad to deg yaw rate/1 -> Yaw rate (deg/s)/1, MinMax Running Resettable/1, Triggered Subsystem2/1(In1), Triggered Subsystem1/1(In1)
  Roll/1 -> rad to deg roll/1
  v/1 -> Lateral speed (m/s)/1, Atan1/1, Sum7/1, Product4/1, Product12/1
  rad to deg roll/1 -> Roll (deg)/1
  Yaw rate/1 -> Multiply/2, Wheelbase/1, rad to deg yaw rate/1
  Hit Crossing/1 -> Triggered Subsystem/Trigger
  Hit Crossing1/1 -> Triggered Subsystem1/Trigger
  rad to deg steer/1 -> Steer (deg)/1
  Hit Crossing3/1 -> Triggered Subsystem2/Trigger
  Triggered Subsystem/1(u) -> Ydisp/1, Compare To Constant/1
  MinMax Running Resettable/1 -> 35%/1, 20%/1
  ISO 2631/1(Frequency weighted accl'n) -> Vertical acceleration (m/s/s)/2, RMS/1(Accel'n)
  Passenger accln/1 -> ISO 2631/1(Passenger accln), Vertical acceleration (m/s/s)/1
  Constant/1 -> Sum3/2
  w/1 -> w (m/s)/1
  p/1 -> p (rad/s)/1
  q/1 -> q (rad/s)/1
  RMS/1(RMS accel'n) -> Triggered Subsystem3/1(RMS accel'n), Vertical acceleration (m/s/s)/3
  RMS/2(Comfort level) -> Comfort level/1
  Triggered Subsystem1/1(Out1) -> Relational Operator/1, Yaw rate (deg/s)/2
  Compare To Constant/1 -> Logical Operator/1
  35%/1 -> Yaw rate (deg/s)/4, Relational Operator/2
  Relational Operator/1 -> Logical Operator/2
  20%/1 -> Relational Operator1/2, Yaw rate (deg/s)/5
  Triggered Subsystem2/1(Out1) -> Relational Operator1/1, Yaw rate (deg/s)/3
  Relational Operator1/1 -> Logical Operator/3
  Logical Operator/1 -> fail_out_yaw_rate/1, Fail/1
  Tevent/1 -> T event (sec)/1, Hit Crossing4/1, Hit Crossing/1, Hit Crossing3/1, Hit Crossing1/1
  Hit Crossing2/1 -> Triggered Subsystem3/Trigger
  Triggered Subsystem3/1(RMS) -> rms accln/1, RMS (m/s/s)/1
  y location1/1 -> Triggered Subsystem/1(In1)
  x location/1 -> Triggered Subsystem5/1(x), Triggered Subsystem4/1(x), x location (m)/1, Hit Crossing2/1, Display/1, X_out/1, x (m)/1, XY Graph/1
  Hit Crossing4/1 -> Triggered Subsystem4/Trigger
  Triggered Subsystem4/1(xs) -> Sum4/2
  u/1 -> [u], Multiply/1, Sum3/1
  Hit Crossing5/1 -> Triggered Subsystem5/Trigger
  Triggered Subsystem5/1(xe) -> Sum4/1
  Sum4/1 -> Braking distance (m)/1
  Pitch/1 -> rad to deg pitch/1
  [u] -> Hit Crossing5/1
  Multiply/1 -> y accl'n/1
  y accl'n/1 -> Sum7/2
  Sum7/1 -> y location1/1
  rad to deg yaw/1 -> Yaw (deg)/1
  Abs/1 -> MinMax Running Resettable1/1
  MinMax Running Resettable1/1 -> Compare To Constant1/1
  Compare To Constant1/1 -> fail_out_body_slip/1, Fail braking/1
  Constant1/1 -> MinMax Running Resettable1/2
  Constant2/1 -> MinMax Running Resettable/2

== system Generic_sedan/Program ==
  Braking trigger : Inport
  Brake switch : Gain  Gain=0
  Decel : Gain  Gain=-0.7
  Gain1 : Gain  Gain=5
  Gain2 : Gain  Gain=2*pi
  No reverse : Saturate  UpperLimit=Inf  LowerLimit=-75/3.6
  Set limit speed : Saturate  UpperLimit=22.4  LowerLimit=0
  Speed request : simulink/Sources/Ramp  slope=0.4*9.8  start=0  InitialOutput=0
  Sum : Sum  Inputs=|++
  Trigonometric Function : Trigonometry
  g : Gain  Gain=9.81
  Extra : Outport
  Speed : Outport  Port=2
  wires:
  g/1 -> No reverse/1
  Set limit speed/1 -> Sum/1
  Trigonometric Function/1 -> Gain1/1
  Gain2/1 -> Trigonometric Function/1
  Brake switch/1 -> Gain2/1, Decel/1
  No reverse/1 -> Sum/2
  Speed request/1 -> Set limit speed/1
  Braking trigger/1 -> Brake switch/1
  Sum/1 -> Speed/1
  Gain1/1 -> Extra/1
  Decel/1 -> g/1

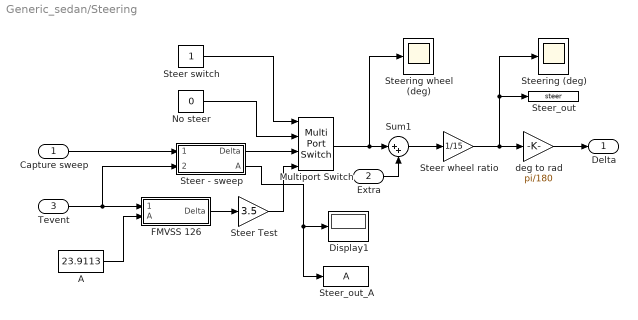
== system Generic_sedan/Steering ==
  Capture sweep : Inport
  Extra : Inport  Port=2
  Tevent : Inport  Port=3
  A : Constant  Value=23.9113
  Display1 : Display
  FMVSS 126 : Subsystem
  Multiport Switch : MultiPortSwitch  SaturateOnIntegerOverflow=off  InputSameDT=off
  No steer : Constant  Value=0
  Steer - sweep : Subsystem
  Steer Test : Gain  Gain=3.5
  Steer switch : Constant
  Steer wheel ratio : Gain  Gain=1/15
  Steer_out : ToWorkspace  VariableName=steer  SaveFormat=Timeseries  SampleTime=-1
      settings: Decimation=3
  Steer_out_A : ToWorkspace  VariableName=A  SaveFormat=Timeseries  SampleTime=-1
      settings: MaxDataPoints=1  Decimation=3
  Steering (deg) : Scope
  Steering wheel (deg) : Scope
  Sum1 : Sum  Inputs=|++
  deg to rad : Gain  Gain=pi/180
  Delta : Outport
  wires:
  Capture sweep/1 -> Steer - sweep/1(Capture)
  Steer wheel ratio/1 -> Steering (deg)/1, Steer_out/1, deg to rad/1
  Steer - sweep/1(Delta) -> Multiport Switch/3
  No steer/1 -> Multiport Switch/2
  Steer Test/1 -> Multiport Switch/4
  Multiport Switch/1 -> Sum1/1, Steering wheel (deg)/1
  Steer switch/1 -> Multiport Switch/1
  Tevent/1 -> Steer - sweep/2(Tevent), FMVSS 126/1(Tevent)
  A/1 -> FMVSS 126/2(A)
  Steer - sweep/2(A) -> Steer_out_A/1, Display1/1
  FMVSS 126/1(Delta) -> Steer Test/1
  Extra/1 -> Sum1/2
  deg to rad/1 -> Delta/1
  Sum1/1 -> Steer wheel ratio/1

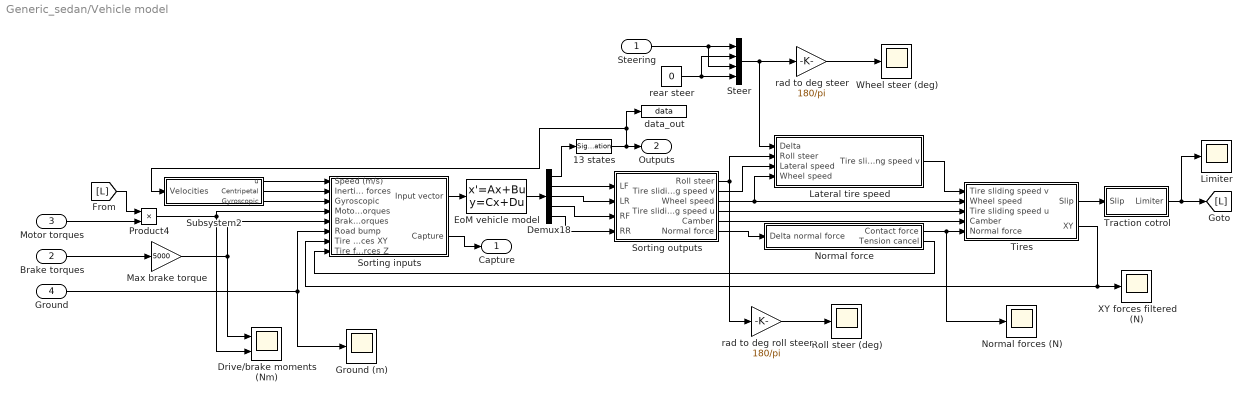
== system Generic_sedan/Vehicle model ==
  Steering : Inport
  Brake torques : Inport  Port=2
  Motor torques : Inport  Port=3
  Ground : Inport  Port=4
  13 states : SignalSpecification  Dimensions=13
  Demux18 : Demux  Outputs=5
  Drive/brake moments (Nm) : Scope  NumInputPorts=2
  EoM vehicle model : StateSpace  A=A  B=B  C=C  D=D  InitialCondition=0
  Ground (m) : Scope
  Lateral tire speed : Subsystem
  Limiter : Scope
  Max brake torque : Gain  Gain=5000
  Normal force : Subsystem
  Normal forces (N) : Scope
  Product4 : Product
  Roll steer (deg) : Scope
  Sorting inputs : Subsystem
  Sorting outputs : Subsystem
  Steer : Mux
  Subsystem2 : Subsystem
  Tires : Subsystem
  Traction cotrol : Subsystem
  Wheel steer (deg) : Scope
  XY forces filtered (N) : Scope
  data_out : ToWorkspace  VariableName=data  SaveFormat=Timeseries  SampleTime=-1
      settings: Decimation=3
  rad to deg roll steer : Gain  Gain=180/pi
  rad to deg steer : Gain  Gain=180/pi
  rear steer : Constant  Value=0
  Capture : Outport
  Outputs : Outport  Port=2
  wires:
  Steering/1 -> Steer/1, Steer/3
  rear steer/1 -> Steer/2, Steer/4
  Subsystem2/1(u) -> Sorting inputs/1(Speed (m/s))
  Sorting outputs/5(Camber) -> Tires/4(Camber)
  EoM vehicle model/1 -> Demux18/1
  Sorting inputs/1(Input vector) -> EoM vehicle model/1
  Demux18/2 -> Sorting outputs/1(LF)
  Demux18/3 -> Sorting outputs/2(LR)
  Demux18/4 -> Sorting outputs/3(RF)
  Demux18/5 -> Sorting outputs/4(RR)
  Subsystem2/2(Centripetal) -> Sorting inputs/2(Inertial forces)
  Sorting outputs/4(Tire sliding speed u) -> Tires/3(Tire sliding speed u)
  Steer/1 -> Lateral tire speed/1(Delta), rad to deg steer/1
  Sorting outputs/1(Roll steer) -> Lateral tire speed/2(Roll steer), rad to deg roll steer/1
  Sorting outputs/2(Tire sliding speed v) -> Lateral tire speed/3(Lateral speed)
  Sorting outputs/6(Normal force) -> Normal force/1(Delta normal force)
  Normal force/2(Tension cancel) -> Sorting inputs/8(Tire forces Z)
  Demux18/1 -> 13 states/1
  rad to deg roll steer/1 -> Roll steer (deg)/1
  rad to deg steer/1 -> Wheel steer (deg)/1
  Motor torques/1 -> Product4/2
  Traction cotrol/1(Limiter) -> [L], Limiter/1
  Tires/1(Slip) -> Traction cotrol/1(Slip)
  Lateral tire speed/1(Tire sliding speed v) -> Tires/1(Tire sliding speed v)
  Sorting outputs/3(Wheel speed) -> Tires/2(Wheel speed), Lateral tire speed/4(Wheel speed)
  Normal force/1(Contact force) -> Normal forces (N)/1, Tires/5(Normal force)
  Tires/2(XY) -> Sorting inputs/7(Tire forces XY), XY forces filtered (N)/1
  Sorting inputs/2(Capture) -> Capture/1
  Brake torques/1 -> Max brake torque/1
  Max brake torque/1 -> Drive/brake moments (Nm)/1, Sorting inputs/5(Brake torques)
  Product4/1 -> Sorting inputs/4(Motor torques), Drive/brake moments (Nm)/2
  Ground/1 -> Ground (m)/1, Sorting inputs/6(Road bump)
  13 states/1 -> Outputs/1, Subsystem2/1(Velocities), data_out/1
  [L] -> Product4/1
  Subsystem2/3(Gyroscopic) -> Sorting inputs/3(Gyroscopic)

== system Generic_sedan/Driver model/Triggered Subsystem ==
  Trigger : TriggerPort  VariantControl=(inherit)
  Constant : Constant
  Out1 : Outport  InitialOutput=0
  wires:
  Constant/1 -> Out1/1

== system Generic_sedan/Driver model/Triggered Subsystem1 ==
  In1 : Inport
  Trigger : TriggerPort  VariantControl=(inherit)
  Constant : Constant
  Out1 : Outport  InitialOutput=0
  Start time : Outport  Port=2  InitialOutput=0
  wires:
  Constant/1 -> Out1/1
  In1/1 -> Start time/1

== system Generic_sedan/Process outputs/ISO 2631 ==
  Passenger accln : Inport
  Hh : TransferFcn  Numerator=[1,0,0 ]  Denominator="[1, sqrt(2)*2*pi*0.4, (2*pi*0.4)^2  ]"
  Hl : TransferFcn  Denominator=[1/(2*pi*100)^2,sqrt(2)/(2*pi*100),1]
  Hs : TransferFcn  Numerator=[1, 2*pi*2.37/0.91, (2*pi*2.37)^2]  Denominator=[1, 2*pi*3.35/0.91, (2*pi*3.35)^2]
  Ht : TransferFcn  Numerator=[1/(2*pi*12.5), 1]  Denominator=[1/(2*pi*12.5)^2, 1/(0.63*2*pi*12.5), 1]
  Frequency weighted accl'n : Outport
  wires:
  Passenger accln/1 -> Hh/1
  Hh/1 -> Hl/1
  Hl/1 -> Ht/1
  Ht/1 -> Hs/1
  Hs/1 -> Frequency weighted accl'n/1

== system Generic_sedan/Process outputs/RMS ==
  Accel'n : Inport
  Clock : Clock
  Compare To Constant : simulink/Logic and Bit Operations/Compare To Constant  relop=>  const=[0, 0.315, 0.5, 0.8, 1.25, 2]  OutDataTypeStr=boolean
  Compare To Constant1 : simulink/Logic and Bit Operations/Compare To Constant  relop=<  const=[0.315, 0.63, 1, 1.6, 2.5, Inf]  OutDataTypeStr=boolean
  Divide : Product  Inputs=*/
  Integrator : Integrator
  Logical Operator : Logic  AllPortsSameDT=off  OutDataTypeStr=boolean
  Math Function : Math  Operator=square
  Saturation : Saturate  UpperLimit=Inf  LowerLimit=1e-9
  Sqrt : Sqrt
  RMS accel'n : Outport
  Comfort level : Outport  Port=2
  wires:
  Accel'n/1 -> Math Function/1
  Math Function/1 -> Integrator/1
  Integrator/1 -> Divide/1
  Saturation/1 -> Divide/2
  Divide/1 -> Sqrt/1
  Logical Operator/1 -> Comfort level/1
  Sqrt/1 -> RMS accel'n/1, Compare To Constant/1, Compare To Constant1/1
  Compare To Constant1/1 -> Logical Operator/2
  Compare To Constant/1 -> Logical Operator/1
  Clock/1 -> Saturation/1

== system Generic_sedan/Process outputs/Triggered Subsystem ==
  In1 : Inport
  Trigger : TriggerPort  VariantControl=(inherit)
  u : Outport
  wires:
  In1/1 -> u/1

== system Generic_sedan/Process outputs/Triggered Subsystem1 ==
  In1 : Inport
  Trigger : TriggerPort  VariantControl=(inherit)
  Out1 : Outport
  wires:
  In1/1 -> Out1/1

== system Generic_sedan/Process outputs/Triggered Subsystem2 ==
  In1 : Inport
  Trigger : TriggerPort  VariantControl=(inherit)
  Out1 : Outport
  wires:
  In1/1 -> Out1/1

== system Generic_sedan/Process outputs/Triggered Subsystem3 ==
  RMS accel'n : Inport
  Trigger : TriggerPort  VariantControl=(inherit)
  RMS : Outport
  wires:
  RMS accel'n/1 -> RMS/1

== system Generic_sedan/Process outputs/Triggered Subsystem4 ==
  x : Inport
  Trigger : TriggerPort  VariantControl=(inherit)
  xs : Outport
  wires:
  x/1 -> xs/1

== system Generic_sedan/Process outputs/Triggered Subsystem5 ==
  x : Inport
  Trigger : TriggerPort  VariantControl=(inherit)
  xe : Outport
  wires:
  x/1 -> xe/1

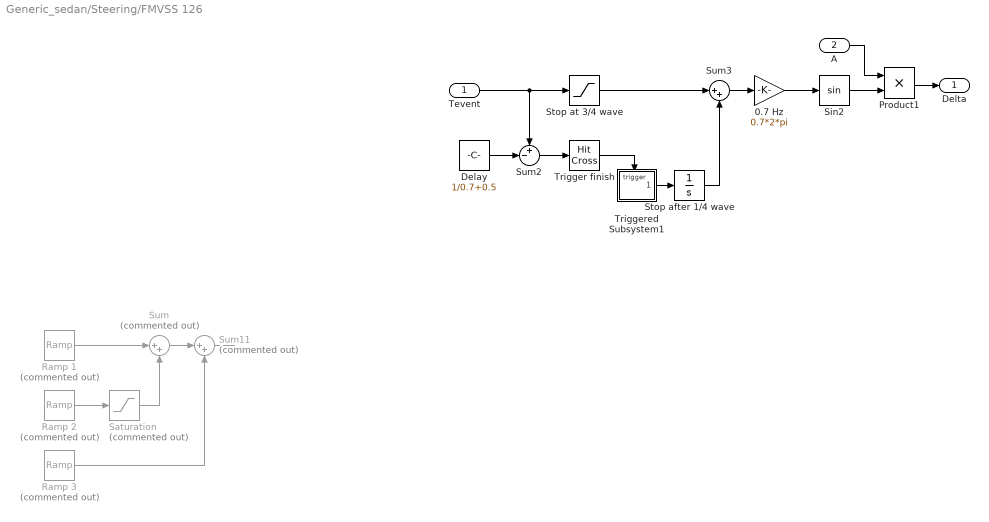
== system Generic_sedan/Steering/FMVSS 126 ==
  Tevent : Inport
  A : Inport  Port=2
  0.7 Hz : Gain  Gain=0.7*2*pi
  Delay : Constant  Value=1/0.7+0.5
  Product1 : Product
  Ramp 1 : simulink/Sources/Ramp  Commented=on  slope=0.7 * 2 * pi  start=10  InitialOutput=0
  Ramp 2 : simulink/Sources/Ramp  Commented=on  slope=-0.7 * 2 * pi  start=10+0.75/0.7  InitialOutput=0
  Ramp 3 : simulink/Sources/Ramp  Commented=on  slope=-0.7 * 2 * pi  start=10+1/0.7 + 0.5  InitialOutput=0
  Saturation : Saturate  Commented=on  UpperLimit=Inf  LowerLimit=-0.5 * 0.7 * 2 * pi
  Sin2 : Trigonometry
  Stop after 1/4 wave : Integrator  LimitOutput=on  UpperSaturationLimit=0.25/0.7
  Stop at 3/4 wave : Saturate  UpperLimit=0.75/0.7  LowerLimit=-Inf
  Sum : Sum  Commented=on  Inputs=|++
  Sum11 : Sum  Commented=on  Inputs=|++
  Sum2 : Sum  Inputs=+-|
  Sum3 : Sum  Inputs=|++
  Trigger finish : HitCross  HitCrossingDirection=rising
  Triggered Subsystem1 : Subsystem  TreatAsAtomicUnit=on
  Delta : Outport
  wires:
  Product1/1 -> Delta/1
  Sin2/1 -> Product1/2
  A/1 -> Product1/1
  Delay/1 -> Sum2/2
  Sum2/1 -> Trigger finish/1
  Trigger finish/1 -> Triggered Subsystem1/Trigger
  Triggered Subsystem1/1(Out1) -> Stop after 1/4 wave/1
  Stop after 1/4 wave/1 -> Sum3/2
  Saturation/1 -> Sum/2
  Ramp 3/1 -> Sum11/2
  Ramp 2/1 -> Saturation/1
  Ramp 1/1 -> Sum/1
  Sum/1 -> Sum11/1
  Sum11/1 -> ?
  0.7 Hz/1 -> Sin2/1
  Tevent/1 -> Sum2/1, Stop at 3/4 wave/1
  Stop at 3/4 wave/1 -> Sum3/1
  Sum3/1 -> 0.7 Hz/1

== system Generic_sedan/Steering/Steer - sweep ==
  Capture : Inport
  Tevent : Inport  Port=2
  13.5 degree : Gain  Gain=13.5
  Saturation : Saturate  UpperLimit=300  LowerLimit=-300
  Steering wheel (deg) : Scope  NumInputPorts=2
  Triggered Subsystem : Subsystem  TreatAsAtomicUnit=on
  Delta : Outport
  A : Outport  Port=2
  wires:
  Saturation/1 -> Steering wheel (deg)/1, Delta/1, Triggered Subsystem/1(In1)
  Triggered Subsystem/1(A) -> Steering wheel (deg)/2, A/1
  Capture/1 -> Triggered Subsystem/Trigger
  13.5 degree/1 -> Saturation/1
  Tevent/1 -> 13.5 degree/1

== system Generic_sedan/Vehicle model/Lateral tire speed ==
  Delta : Inport
  Roll steer : Inport  Port=2
  Lateral speed : Inport  Port=3
  Wheel speed : Inport  Port=4
  Product4 : Product
  Sum10 : Sum  Inputs=++|
  Sum9 : Sum  Inputs=|-+
  Tire sliding speed v : Outport
  wires:
  Sum10/1 -> Product4/1
  Product4/1 -> Sum9/1
  Delta/1 -> Sum10/1
  Sum9/1 -> Tire sliding speed v/1
  Lateral speed/1 -> Sum9/2
  Roll steer/1 -> Sum10/2
  Wheel speed/1 -> Product4/2

== system Generic_sedan/Vehicle model/Normal force ==
  Delta normal force : Inport
  Saturation : Saturate  UpperLimit=Inf  LowerLimit=1e-6
  Sum1 : Sum  Inputs=|-+
  Sum8 : Sum  Inputs=+-|
  Z0 : Constant  Value=Z0
  Contact force : Outport
  Tension cancel : Outport  Port=2
  wires:
  Sum8/1 -> Tension cancel/1
  Sum1/1 -> Saturation/1, Sum8/2
  Z0/1 -> Sum1/2
  Delta normal force/1 -> Sum1/1
  Saturation/1 -> Contact force/1, Sum8/1

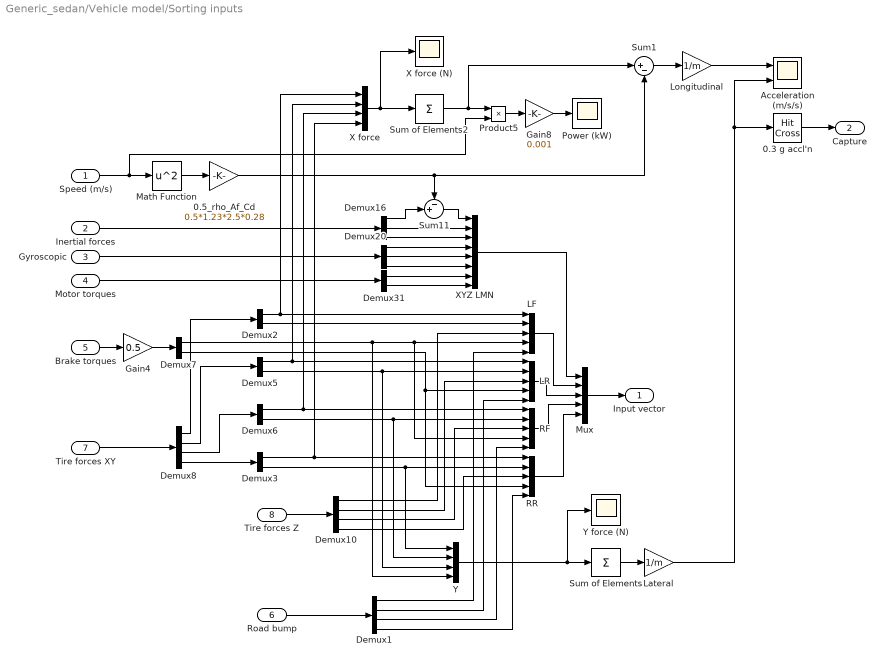
== system Generic_sedan/Vehicle model/Sorting inputs ==
  Speed (m/s) : Inport
  Inertial forces : Inport  Port=2
  Gyroscopic : Inport  Port=3
  Motor torques : Inport  Port=4
  Brake torques : Inport  Port=5
  Road bump : Inport  Port=6
  Tire forces XY : Inport  Port=7
  Tire forces Z : Inport  Port=8
  0.3 g accl'n : HitCross  HitCrossingOffset=0.3*9.81  HitCrossingDirection=rising
  0.5_rho_Af_Cd : Gain  Gain=0.5*1.23*2.5*0.28
  Acceleration (m/s/s) : Scope  NumInputPorts=2
  Demux1 : Demux
  Demux10 : Demux
  Demux16 : Demux  Outputs=3
  Demux{2..3,5..7,31} (6 alike) : Demux  Outputs=2
  Demux20 : Demux  Outputs=3
  Demux8 : Demux
  Gain4 : Gain  Gain=0.5
  Gain8 : Gain  Gain=0.001
  LF : Mux  Inputs=5
  LR : Mux  Inputs=5
  Lateral : Gain  Gain=1/m
  Longitudinal : Gain  Gain=1/m
  Math Function : Math  Operator=square
  Mux : Mux  Inputs=5
  Power (kW) : Scope
  Product5 : Product
  RF : Mux  Inputs=5
  RR : Mux  Inputs=5
  Sum of Elements : Sum  Inputs=+
  Sum of Elements2 : Sum  Inputs=+
  Sum1 : Sum  Inputs=|+-
  Sum11 : Sum  Inputs=-+|
  X force : Mux
  X force (N) : Scope
  XYZ LMN : Mux  Inputs=8
  Y : Mux
  Y force (N) : Scope
  Input vector : Outport
  Capture : Outport  Port=2
  wires:
  Demux16/3 -> XYZ LMN/3
  RF/1 -> Mux/4
  Demux20/2 -> XYZ LMN/5
  Demux10/4 -> RR/3
  Demux7/2 -> RR/4, LR/4
  Mux/1 -> Input vector/1
  Demux16/1 -> Sum11/2
  RR/1 -> Mux/5
  Tire forces Z/1 -> Demux10/1
  Demux6/1 -> RF/1, X force/3
  LF/1 -> Mux/2
  Demux10/3 -> RF/3
  LR/1 -> Mux/3
  Sum11/1 -> XYZ LMN/1
  Tire forces XY/1 -> Demux8/1
  0.5_rho_Af_Cd/1 -> Sum11/1, Sum1/2
  Demux3/1 -> RR/1, X force/4
  Demux6/2 -> RF/2, Y/2
  Demux5/2 -> LR/2, Y/3
  Motor torques/1 -> Demux31/1
  X force/1 -> Sum of Elements2/1, X force (N)/1
  Demux8/4 -> Demux3/1
  Inertial forces/1 -> Demux16/1
  Demux5/1 -> LR/1, X force/2
  Demux31/2 -> XYZ LMN/8
  Demux8/3 -> Demux6/1
  Demux8/2 -> Demux5/1
  Gyroscopic/1 -> Demux20/1
  Demux20/1 -> XYZ LMN/4
  Demux16/2 -> XYZ LMN/2
  Demux10/2 -> LR/3
  Demux3/2 -> RR/2, Y/1
  Demux20/3 -> XYZ LMN/6
  Demux7/1 -> RF/4, LF/4, Y/4
  Gain4/1 -> Demux7/1
  Demux2/2 -> LF/2
  Demux31/1 -> XYZ LMN/7
  Demux8/1 -> Demux2/1
  Demux2/1 -> LF/1, X force/1
  Brake torques/1 -> Gain4/1
  XYZ LMN/1 -> Mux/1
  Demux10/1 -> LF/3
  Gain8/1 -> Power (kW)/1
  Product5/1 -> Gain8/1
  Math Function/1 -> 0.5_rho_Af_Cd/1
  Speed (m/s)/1 -> Math Function/1, Product5/2
  Y/1 -> Sum of Elements/1, Y force (N)/1
  Sum of Elements2/1 -> Sum1/1, Product5/1
  Sum of Elements/1 -> Lateral/1
  Longitudinal/1 -> Acceleration (m/s/s)/1
  Lateral/1 -> Acceleration (m/s/s)/2, 0.3 g accl'n/1
  Sum1/1 -> Longitudinal/1
  Demux1/1 -> LF/5
  Demux1/2 -> LR/5
  Demux1/3 -> RF/5
  Road bump/1 -> Demux1/1
  Demux1/4 -> RR/5
  0.3 g accl'n/1 -> Capture/1

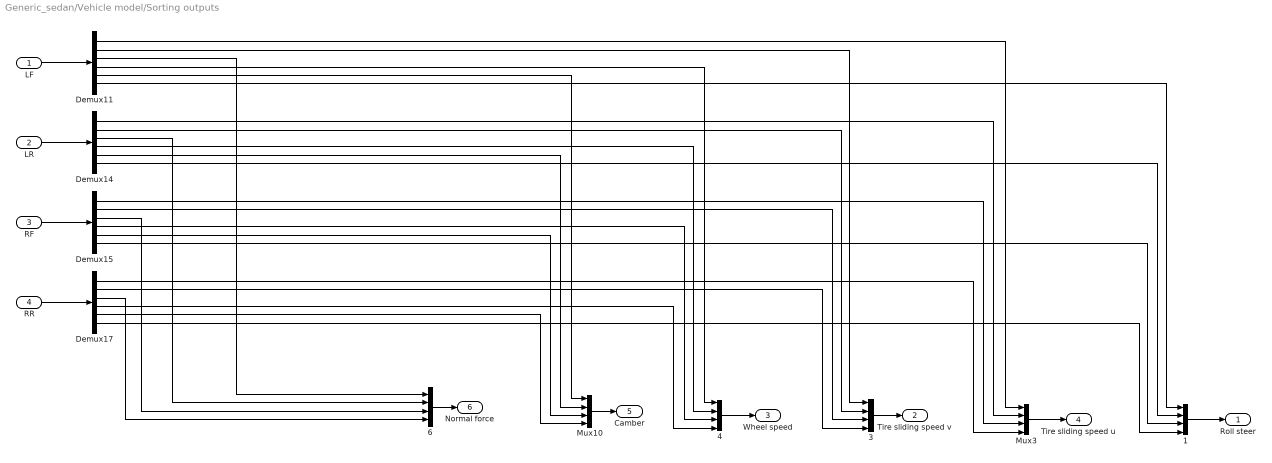
== system Generic_sedan/Vehicle model/Sorting outputs ==
  LF : Inport
  LR : Inport  Port=2
  RF : Inport  Port=3
  RR : Inport  Port=4
  {1,3..4,6} (4 alike) : Mux
  Demux{11,14..15,17} (4 alike) : Demux  Outputs=6
  Mux10 : Mux
  Mux3 : Mux
  Roll steer : Outport
  Tire sliding speed v : Outport  Port=2
  Wheel speed : Outport  Port=3
  Tire sliding speed u : Outport  Port=4
  Camber : Outport  Port=5
  Normal force : Outport  Port=6
  wires:
  6/1 -> Normal force/1
  Demux15/4 -> 4/3
  Demux11/4 -> 4/1
  Demux14/3 -> 6/2
  Demux14/4 -> 4/2
  Demux11/1 -> Mux3/1
  Demux14/1 -> Mux3/2
  Demux11/6 -> 1/1
  Demux15/1 -> Mux3/3
  Demux15/3 -> 6/3
  Demux17/3 -> 6/4
  Demux14/5 -> Mux10/2
  1/1 -> Roll steer/1
  Demux14/6 -> 1/2
  Mux10/1 -> Camber/1
  3/1 -> Tire sliding speed v/1
  Demux15/2 -> 3/3
  Mux3/1 -> Tire sliding speed u/1
  Demux17/4 -> 4/4
  LR/1 -> Demux14/1
  RF/1 -> Demux15/1
  RR/1 -> Demux17/1
  Demux15/6 -> 1/3
  Demux17/2 -> 3/4
  LF/1 -> Demux11/1
  Demux14/2 -> 3/2
  Demux11/5 -> Mux10/1
  Demux11/2 -> 3/1
  Demux17/1 -> Mux3/4
  Demux17/6 -> 1/4
  4/1 -> Wheel speed/1
  Demux11/3 -> 6/1
  Demux17/5 -> Mux10/4
  Demux15/5 -> Mux10/3

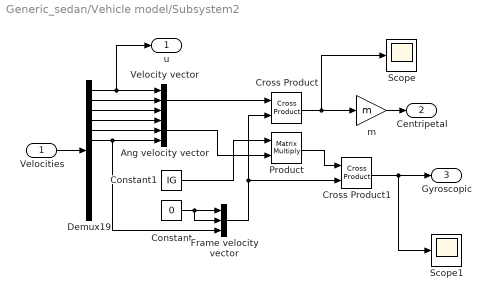
== system Generic_sedan/Vehicle model/Subsystem2 ==
  Velocities : Inport
  Ang velocity vector : Mux  Inputs=3
  Constant : Constant  Value=0
  Constant1 : Constant  Value=IG
  Cross Product : matrix_library/Cross Product
  Cross Product1 : matrix_library/Cross Product
  Demux19 : Demux  Outputs=13
  Frame velocity vector : Mux  Inputs=3
  Product : Product  Multiplication=Matrix(*)
  Scope : Scope
  Scope1 : Scope
  Velocity vector : Mux  Inputs=3
  m : Gain  Gain=m
  u : Outport
  Centripetal : Outport  Port=2
  Gyroscopic : Outport  Port=3
  wires:
  Demux19/2 -> Velocity vector/2
  Cross Product/1 -> Scope/1, m/1
  Demux19/3 -> Velocity vector/3
  Demux19/5 -> Ang velocity vector/2
  Demux19/6 -> Ang velocity vector/3, Frame velocity vector/3
  Frame velocity vector/1 -> Cross Product1/2, Cross Product/2
  Demux19/4 -> Ang velocity vector/1
  Demux19/1 -> u/1, Velocity vector/1
  Velocity vector/1 -> Cross Product/1
  m/1 -> Centripetal/1
  Velocities/1 -> Demux19/1
  Constant/1 -> Frame velocity vector/2, Frame velocity vector/1
  Constant1/1 -> Product/1
  Ang velocity vector/1 -> Product/2
  Product/1 -> Cross Product1/1
  Cross Product1/1 -> Gyroscopic/1, Scope1/1
